simulink model "Example"  (R2016a)
settings: Solver=FixedStepAuto  StartTime=0.0  StopTime=EndTime  FixedStep=SampleTime  RelTol=1e-3
values from neighbouring files (symbols this model uses):
  A1_IC = pi/4    (= 0.785398163397)    [LaserBeamStability_CommandScript.m]
  A2_IC = pi/4    (= 0.785398163397)    [LaserBeamStability_CommandScript.m]
  A3_IC = pi/4    (= 0.785398163397)    [LaserBeamStability_CommandScript.m]
  A4_IC = pi/4    (= 0.785398163397)    [LaserBeamStability_CommandScript.m]
  ActArm = 3.85    [LaserBeamStability_CommandScript.m]
  b12 = d(14)-d(14)*d(15)/f(2)+d(15)    [LaserBeamStability_CommandScript.m]
  b34 = d(18)-(d(18)*d(19))/f(4)+d(19)    [LaserBeamStability_CommandScript.m]
  c12 = pi/2-2*Beta(2)    [LaserBeamStability_CommandScript.m]
  c34 = pi/2-2*Beta(4)    [LaserBeamStability_CommandScript.m]
  EndTime = 1    [LaserBeamStability_CommandScript.m]
  g12 = d(13)-d(13)*d(12)/f(1)+d(12)    [LaserBeamStability_CommandScript.m]
  g34 = d(17)-(d(17)*d(16))/f(3)+d(16)    [LaserBeamStability_CommandScript.m]
  h12 = pi/2-2*Beta(1)    [LaserBeamStability_CommandScript.m]
  h34 = pi/2-2*Beta(3)    [LaserBeamStability_CommandScript.m]
  n_BS = 1.52    [LaserBeamStability_CommandScript.m]
  n_FS = 1.00    (= 1)    [LaserBeamStability_CommandScript.m]
  NuetralPoint = (Maximum_Extension-Minimum_Extension)/2    (= 6.25)    [LaserBeamStability_CommandScript.m]
  Optical_Plane_1_Command = [0 0]    [LaserBeamStability_CommandScript.m]
  SampleTime = 1/10    (= 0.1)    [LaserBeamStability_CommandScript.m]
  Sensor12Matx = [a12+b12/d(6) -b12/d(6); g12/d(6) e12-g12/d(6)]    [LaserBeamStability_CommandScript.m]
  Sensor34Matx = [a34+b34/d(10) -b34/d(10); g34/d(10) e34-g34/d(10)]    [LaserBeamStability_CommandScript.m]
  SocketID = TCP_ConnectToServer(IP_ADD, Port, TimeOut)    [LaserBeamStability_CommandScript.m]
  t12 = 2.5    [LaserBeamStability_CommandScript.m]
  t34 = 2.5    [LaserBeamStability_CommandScript.m]
  Target_Command = [0 0]    [LaserBeamStability_CommandScript.m]
undefined symbols (not defined in the file or in its folder): A, Beta, D, d, f, l, positioner, Td, TLense
libraries: simulink x1
settings Model: Creator=Justin  LastModifiedBy=Justin
settings SolverCC: ZeroCrossControl=EnableAll  ZeroCrossAlgorithm=Adaptive

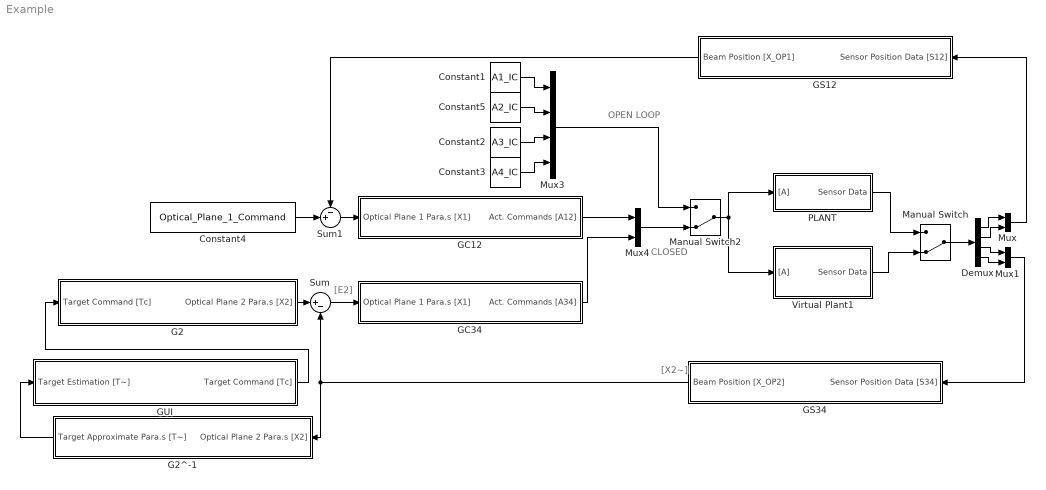
== system Example ==
  note: CLOSED
  note: OPEN LOOP
  note: [X2~]
  note: [E2]
  Constant1 : Constant  Value=A1_IC
  Constant2 : Constant  Value=A3_IC
  Constant3 : Constant  Value=A4_IC
  Constant4 : Constant  Value=Optical_Plane_1_Command
  Constant5 : Constant  Value=A2_IC
  Demux : Demux
  G2 : Subsystem
  G2^-1 : Subsystem
  GC12 : Subsystem
  GC34 : Subsystem
  GS12 : Subsystem
  GS34 : Subsystem
  GUI : Subsystem
  Manual Switch : ManualSwitch  CurrentSetting=0
  Manual Switch2 : ManualSwitch  CurrentSetting=0
  Mux : Mux  Inputs=2
  Mux1 : Mux  Inputs=2
  Mux3 : Mux
  Mux4 : Mux  Inputs=2
  PLANT : Subsystem
  Sum : Sum  Inputs=|+-
  Sum1 : Sum  Inputs=-+|
  Virtual Plant1 : Subsystem
  wires:
  G2/1(Optical Plane 2 Para.s [X2]) -> Sum/1
  G2^-1/1(Target Approximate Para.s [T~]) -> GUI/1(Target Estimation [T~])
  GUI/1(Target Command [Tc]) -> G2/1(Target Command [Tc])
  PLANT/1(Sensor Data) -> Manual Switch/1
  Demux/1 -> Mux/1
  Demux/2 -> Mux/2
  Demux/3 -> Mux1/1
  Demux/4 -> Mux1/2
  Mux/1 -> GS12/1(Sensor Position Data [S12])
  Mux1/1 -> GS34/1(Sensor Position Data [S34])
  Sum/1 -> GC34/1(Optical Plane 1 Para.s [X1])
  GC34/1(Act. Commands [A34]) -> Mux4/2
  GS34/1(Beam Position [X_OP2]) -> G2^-1/1(Optical Plane 2 Para.s [X2]), Sum/2
  Sum1/1 -> GC12/1(Optical Plane 1 Para.s [X1])
  GS12/1(Beam Position [X_OP1]) -> Sum1/1
  Constant5/1 -> Mux3/2
  Constant1/1 -> Mux3/1
  GC12/1(Act. Commands [A12]) -> Mux4/1
  Virtual Plant1/1(Sensor Data) -> Manual Switch/2
  Manual Switch/1 -> Demux/1
  Constant2/1 -> Mux3/3
  Constant3/1 -> Mux3/4
  Mux4/1 -> Manual Switch2/2
  Mux3/1 -> Manual Switch2/1
  Manual Switch2/1 -> Virtual Plant1/1("[A]"), PLANT/1("[A]")
  Constant4/1 -> Sum1/2

== system Example/G2 ==
  Target Command [Tc] : Inport
  Beam Pass 3 Inv : Subsystem
  Beam Pass 4 Inv : Subsystem
  l10 inv : Gain  Gain=([1 d(10); 0 1])^-1  Multiplication=Matrix(K*u)
  l11 inv : Gain  Gain=([1 d(11); 0 1])^-1  Multiplication=Matrix(K*u)
  l9 inv : Gain  Gain=([1 d(9); 0 1])^-1  Multiplication=Matrix(K*u)
  Optical Plane 2 Para.s [X2] : Outport
  wires:
  Target Command [Tc]/1 -> l11 inv/1
  l11 inv/1 -> Beam Pass 4 Inv/1(Passed Parameters)
  Beam Pass 4 Inv/1("Approximated Incoming Parameters ") -> l10 inv/1
  l10 inv/1 -> Beam Pass 3 Inv/1(Passed Parameters)
  Beam Pass 3 Inv/1("Approximated Incoming Parameters ") -> l9 inv/1
  l9 inv/1 -> Optical Plane 2 Para.s [X2]/1

== system Example/G2^-1 ==
  Optical Plane 2 Para.s [X2] : Inport
  Beam Pass 3 : Subsystem
  Beam Pass 4 : Subsystem
  l(10) : Gain  Gain=([1 d(10); 0 1])  Multiplication=Matrix(K*u)
  l(11) : Gain  Gain=([1 d(11); 0 1])  Multiplication=Matrix(K*u)
  l(9) : Gain  Gain=([1 d(9); 0 1])  Multiplication=Matrix(K*u)
  Target Approximate Para.s [T~] : Outport
  wires:
  Optical Plane 2 Para.s [X2]/1 -> l(9)/1
  l(11)/1 -> Target Approximate Para.s [T~]/1
  l(9)/1 -> Beam Pass 3/1(Approximated Optical Plane 2 Parameters)
  Beam Pass 3/1("Approximated Target Parameters ") -> l(10)/1
  l(10)/1 -> Beam Pass 4/1(Approximated Optical Plane 2 Parameters)
  Beam Pass 4/1("Approximated Target Parameters ") -> l(11)/1

== system Example/GC12 ==
  Optical Plane 1 Para.s [X1] : Inport
  IC2 : InitialCondition  Value=[A1_IC A2_IC]
  Sum : Sum  Inputs=|++
  Transport^-1 : Subsystem
  Unit Delay2 : UnitDelay  InitialCondition=[A1_IC A2_IC]  SampleTime=SampleTime
  "[Nu]^-1" : Subsystem
  Act. Commands [A12] : Outport
  wires:
  Optical Plane 1 Para.s [X1]/1 -> Transport^-1/1(Optical Plane 1 Para.s [X1])
  "[Nu]^-1"/1("[A_12]") -> Sum/1
  Sum/1 -> IC2/1
  Transport^-1/1("[E_A2']") -> "[Nu]^-1"/1("[E_A2']")
  IC2/1 -> Unit Delay2/1, Act. Commands [A12]/1
  Unit Delay2/1 -> "[Nu]^-1"/2("[A_12]z^-1"), Sum/2

== system Example/GC34 ==
  Optical Plane 1 Para.s [X1] : Inport
  Demux : Demux  Outputs=2
  IC2 : InitialCondition  Value=[A1_IC A2_IC]
  Mux : Mux  Inputs=2
  Sum : Sum  Inputs=|++
  Transport^-1 : Subsystem
  Unit Delay : UnitDelay  InitialCondition=A1_IC  SampleTime=SampleTime
  Unit Delay1 : UnitDelay  InitialCondition=A2_IC  SampleTime=SampleTime
  "[Nu]^-1" : Subsystem
  Act. Commands [A34] : Outport
  wires:
  IC2/1 -> Act. Commands [A34]/1, Demux/1
  Demux/2 -> Unit Delay1/1
  Demux/1 -> Unit Delay/1
  Unit Delay1/1 -> Mux/2
  Unit Delay/1 -> Mux/1
  Transport^-1/1("[E_A2']") -> "[Nu]^-1"/1("[E_A2']")
  Mux/1 -> Sum/2, "[Nu]^-1"/2("[A_12]z^-1")
  Sum/1 -> IC2/1
  "[Nu]^-1"/1("[A_12]") -> Sum/1
  Optical Plane 1 Para.s [X1]/1 -> Transport^-1/1(Optical Plane 1 Para.s [X1])

== system Example/GS12 ==
  note: Theta op1
  note: rop1
  note: R_S2
  note: R_S1
  note: rl6'
  note: rop1
  Sensor Position Data [S12] : Inport
  Constant1 : Constant  Value=b12*c12
  Constant2 : Constant  Value=d(6)
  Constant6 : Constant  Value=g12*h12
  Demux : Demux  Outputs=2
  Demux1 : Demux  Outputs=2
  Gain : Gain  Gain=Sensor12Matx^-1  Multiplication=Matrix(K*u)
  Mux : Mux  Inputs=2
  Mux1 : Mux  Inputs=2
  Product : Product  Inputs=*/
  Sum : Sum  Inputs=|+-
  Sum1 : Sum  Inputs=-+|
  Sum2 : Sum  Inputs=+-|
  Beam Position [X_OP1] : Outport
  wires:
  Product/1 -> Mux/2
  Constant2/1 -> Product/2
  Sum2/1 -> Product/1
  Demux1/1 -> Sum2/1
  Demux1/2 -> Mux/1, Sum2/2
  Sum/1 -> Mux1/2
  Sum1/1 -> Mux1/1
  Mux1/1 -> Gain/1
  Constant6/1 -> Sum/2
  Constant1/1 -> Sum1/1
  Demux/1 -> Sum/1
  Demux/2 -> Sum1/2
  Gain/1 -> Demux1/1
  Sensor Position Data [S12]/1 -> Demux/1
  Mux/1 -> Beam Position [X_OP1]/1

== system Example/GS34 ==
  note: rop2
  note: rl10'
  note: R_S3
  note: R_S4
  note: rop2
  note: Theta op2
  Sensor Position Data [S34] : Inport
  Constant1 : Constant  Value=b34*c34
  Constant2 : Constant  Value=d(10)
  Constant6 : Constant  Value=g34*h34
  Demux : Demux  Outputs=2
  Demux1 : Demux  Outputs=2
  Gain : Gain  Gain=Sensor34Matx^-1  Multiplication=Matrix(K*u)
  Mux : Mux  Inputs=2
  Mux1 : Mux  Inputs=2
  Product : Product  Inputs=*/
  Sum : Sum  Inputs=|+-
  Sum1 : Sum  Inputs=-+|
  Sum2 : Sum  Inputs=+-|
  Beam Position [X_OP2] : Outport
  wires:
  Mux/1 -> Beam Position [X_OP2]/1
  Sensor Position Data [S34]/1 -> Demux/1
  Gain/1 -> Demux1/1
  Demux/2 -> Sum1/2
  Demux/1 -> Sum/1
  Constant1/1 -> Sum1/1
  Constant6/1 -> Sum/2
  Mux1/1 -> Gain/1
  Sum1/1 -> Mux1/1
  Sum/1 -> Mux1/2
  Demux1/2 -> Sum2/2, Mux/1
  Demux1/1 -> Sum2/1
  Sum2/1 -> Product/1
  Constant2/1 -> Product/2
  Product/1 -> Mux/2

== system Example/GUI ==
  Target Estimation [T~] : Inport
  Constant : Constant  Value=Target_Command(1)
  Constant1 : Constant  Value=Target_Command(2)
  Mux : Mux  Inputs=2
  "Target Approximation Scope " : Scope
  To Workspace : ToWorkspace  VariableName=Target_Estimation  SaveFormat=Timeseries  SampleTime=-1
  Target Command [Tc] : Outport
  wires:
  Target Estimation [T~]/1 -> To Workspace/1, "Target Approximation Scope "/1
  Mux/1 -> Target Command [Tc]/1
  Constant/1 -> Mux/1
  Constant1/1 -> Mux/2

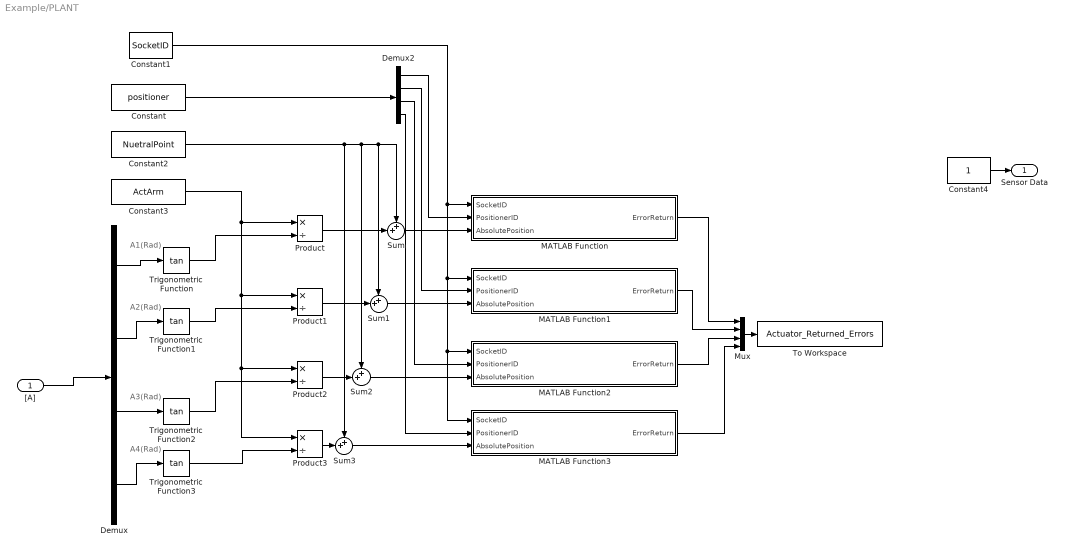
== system Example/PLANT ==
  note: A1(Rad)
  note: A2(Rad)
  note: A3(Rad)
  note: A4(Rad)
  "[A]" : Inport
  Constant : Constant  Value=positioner
  Constant1 : Constant  Value=SocketID
  Constant2 : Constant  Value=NuetralPoint
  Constant3 : Constant  Value=ActArm
  Constant4 : Constant
  Demux : Demux
  Demux2 : Demux
  MATLAB Function : MATLAB Function  TreatAsAtomicUnit=on
  MATLAB Function1 : MATLAB Function  TreatAsAtomicUnit=on
  MATLAB Function2 : MATLAB Function  TreatAsAtomicUnit=on
  MATLAB Function3 : MATLAB Function  TreatAsAtomicUnit=on
  Mux : Mux
  Product{,1..3} (4 alike) : Product  Inputs=*/
  Sum{,1..3} (4 alike) : Sum  Inputs=++|
  To Workspace : ToWorkspace  VariableName=Actuator_Returned_Errors  SaveFormat=Timeseries  SampleTime=-1
  Trigonometric Function{,1..3} (4 alike) : Trigonometry  Operator=tan
  Sensor Data : Outport
  wires:
  "[A]"/1 -> Demux/1
  Constant/1 -> Demux2/1
  Demux2/1 -> MATLAB Function/2(PositionerID)
  Demux2/2 -> MATLAB Function1/2(PositionerID)
  Demux2/3 -> MATLAB Function2/2(PositionerID)
  Demux2/4 -> MATLAB Function3/2(PositionerID)
  Constant1/1 -> MATLAB Function3/1(SocketID), MATLAB Function2/1(SocketID), MATLAB Function1/1(SocketID), MATLAB Function/1(SocketID)
  Sum/1 -> MATLAB Function/3(AbsolutePosition)
  Demux/1 -> Trigonometric Function/1
  Demux/2 -> Trigonometric Function1/1
  Demux/4 -> Trigonometric Function3/1
  Product/1 -> Sum/2
  Product1/1 -> Sum1/2
  Sum1/1 -> MATLAB Function1/3(AbsolutePosition)
  Constant2/1 -> Sum2/1, Sum1/1, Sum/1, Sum3/1
  Sum2/1 -> MATLAB Function2/3(AbsolutePosition)
  Sum3/1 -> MATLAB Function3/3(AbsolutePosition)
  Product3/1 -> Sum3/2
  Product2/1 -> Sum2/2
  Constant3/1 -> Product3/1, Product2/1, Product1/1, Product/1
  Trigonometric Function3/1 -> Product3/2
  Trigonometric Function2/1 -> Product2/2
  Trigonometric Function1/1 -> Product1/2
  Trigonometric Function/1 -> Product/2
  Mux/1 -> To Workspace/1
  MATLAB Function/1(ErrorReturn) -> Mux/1
  MATLAB Function1/1(ErrorReturn) -> Mux/2
  MATLAB Function2/1(ErrorReturn) -> Mux/3
  MATLAB Function3/1(ErrorReturn) -> Mux/4
  Constant4/1 -> Sensor Data/1
  Demux/3 -> Trigonometric Function2/1

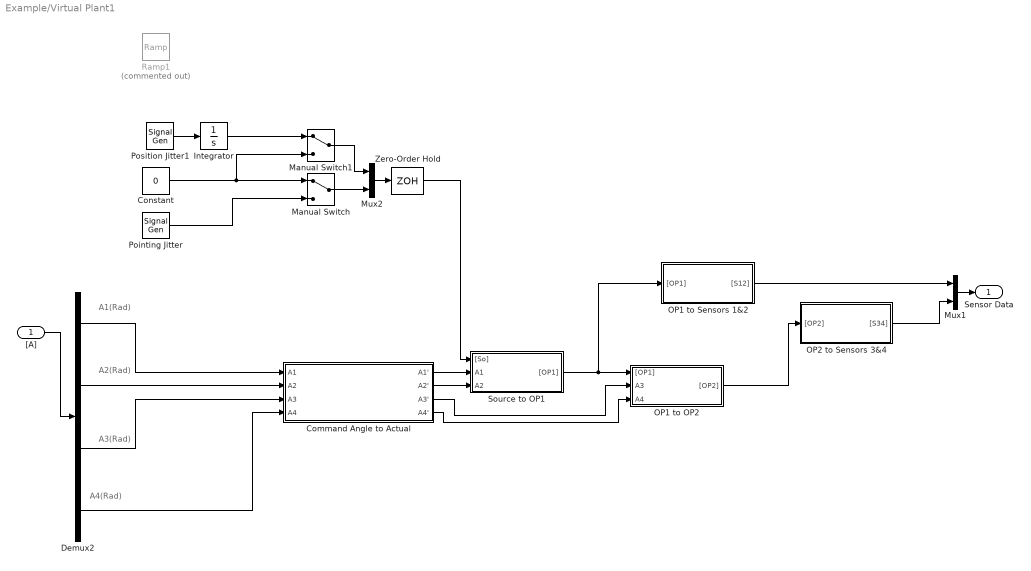
== system Example/Virtual Plant1 ==
  note: A4(Rad)
  note: A3(Rad)
  note: A2(Rad)
  note: A1(Rad)
  "[A]" : Inport
  Command Angle to Actual : Subsystem
  Constant : Constant  Value=0
  Demux2 : Demux
  Integrator : Integrator
  Manual Switch : ManualSwitch
  Manual Switch1 : ManualSwitch
  Mux1 : Mux  Inputs=2
  Mux2 : Mux  Inputs=2
  OP1 to OP2 : Subsystem
  OP1 to Sensors 1&2 : Subsystem
  OP2 to Sensors 3&4 : Subsystem
  Pointing Jitter : SignalGenerator  Amplitude=0.001  Frequency=1/EndTime
  Position Jitter1 : SignalGenerator  WaveForm=random  Amplitude=-0.5  Frequency=5/EndTime
  Ramp1 : simulink/Sources/Ramp  Commented=on  slope=A/EndTime  start=0  X0=0
  Source to OP1 : Subsystem
  Zero-Order Hold : ZeroOrderHold  SampleTime=SampleTime
  Sensor Data : Outport
  wires:
  Pointing Jitter/1 -> Manual Switch/2
  Constant/1 -> Manual Switch1/2, Manual Switch/1
  Manual Switch1/1 -> Mux2/1
  Manual Switch/1 -> Mux2/2
  Mux2/1 -> Zero-Order Hold/1
  OP2 to Sensors 3&4/1("[S34]") -> Mux1/2
  OP1 to OP2/1("[OP2]") -> OP2 to Sensors 3&4/1("[OP2]")
  OP1 to Sensors 1&2/1("[S12]") -> Mux1/1
  Mux1/1 -> Sensor Data/1
  Source to OP1/1("[OP1]") -> OP1 to OP2/1("[OP1]"), OP1 to Sensors 1&2/1("[OP1]")
  Command Angle to Actual/1(A1') -> Source to OP1/2(A1)
  Command Angle to Actual/2(A2') -> Source to OP1/3(A2)
  Command Angle to Actual/3(A3') -> OP1 to OP2/2(A3)
  Command Angle to Actual/4(A4') -> OP1 to OP2/3(A4)
  Demux2/1 -> Command Angle to Actual/1(A1)
  Demux2/2 -> Command Angle to Actual/2(A2)
  Demux2/3 -> Command Angle to Actual/3(A3)
  Demux2/4 -> Command Angle to Actual/4(A4)
  "[A]"/1 -> Demux2/1
  Zero-Order Hold/1 -> Source to OP1/1("[So]")
  Position Jitter1/1 -> Integrator/1
  Integrator/1 -> Manual Switch1/1

== system Example/G2/Beam Pass 3 Inv ==
  note: r'
  note: theta'
  note: r
  note: Theta
  Passed Parameters : Inport
  Demux : Demux  Outputs=2
  Mux : Mux  Inputs=2
  Sine : Trigonometry
  Snell Ratio : Gain  Gain=n_FS/n_BS  Multiplication=Matrix(K*u)
  Sum : Sum  Inputs=|+-
  Sum1 : Sum  Inputs=|+-
  Tangent : Trigonometry  Operator=tan
  Thickness Offset 1 : Gain  Gain=D(3)*cos(Beta(3))
  Thickness Offset 2 : Constant  Value=D(3)*sin(Beta(3))
  "Approximated Incoming Parameters " : Outport
  wires:
  Thickness Offset 2/1 -> Sum1/2
  Thickness Offset 1/1 -> Sum1/1
  Tangent/1 -> Thickness Offset 1/1
  Snell Ratio/1 -> Tangent/1
  Sine/1 -> Snell Ratio/1
  Demux/1 -> Sum/1
  Demux/2 -> Sine/1, Mux/2
  Sum/1 -> Mux/1
  Mux/1 -> "Approximated Incoming Parameters "/1
  Sum1/1 -> Sum/2
  Passed Parameters/1 -> Demux/1

== system Example/G2/Beam Pass 4 Inv ==
  note: Theta
  note: r
  note: theta'
  note: r'
  Passed Parameters : Inport
  Demux : Demux  Outputs=2
  Mux : Mux  Inputs=2
  Sine : Trigonometry
  Snell Ratio : Gain  Gain=n_FS/n_BS
  Sum : Sum  Inputs=|+-
  Sum1 : Sum  Inputs=|+-
  Tangent : Trigonometry  Operator=tan
  Thickness Offset 1 : Gain  Gain=D(4)*cos(Beta(4))
  Thickness Offset 2 : Constant  Value=D(4)*sin(Beta(4))
  "Approximated Incoming Parameters " : Outport
  wires:
  Passed Parameters/1 -> Demux/1
  Sum1/1 -> Sum/2
  Mux/1 -> "Approximated Incoming Parameters "/1
  Sum/1 -> Mux/1
  Demux/2 -> Mux/2, Sine/1
  Demux/1 -> Sum/1
  Sine/1 -> Snell Ratio/1
  Snell Ratio/1 -> Tangent/1
  Tangent/1 -> Thickness Offset 1/1
  Thickness Offset 1/1 -> Sum1/1
  Thickness Offset 2/1 -> Sum1/2

== system Example/G2^-1/Beam Pass 3 ==
  Approximated Optical Plane 2 Parameters : Inport
  Demux : Demux  Outputs=2
  Mux : Mux  Inputs=2
  Sine : Trigonometry
  Snell Ratio : Gain  Gain=n_FS/n_BS
  Sum : Sum  Inputs=|++
  Sum1 : Sum  Inputs=|+-
  Tangent : Trigonometry  Operator=tan
  Thickness Offset 1 : Gain  Gain=D(3)*cos(Beta(3))
  Thickness Offset 2 : Constant  Value=D(3)*sin(Beta(3))
  "Approximated Target Parameters " : Outport
  wires:
  Approximated Optical Plane 2 Parameters/1 -> Demux/1
  Mux/1 -> "Approximated Target Parameters "/1
  Demux/1 -> Sum/1
  Sum/1 -> Mux/1
  Sum1/1 -> Sum/2
  Demux/2 -> Sine/1, Mux/2
  Snell Ratio/1 -> Tangent/1
  Sine/1 -> Snell Ratio/1
  Tangent/1 -> Thickness Offset 1/1
  Thickness Offset 1/1 -> Sum1/1
  Thickness Offset 2/1 -> Sum1/2

== system Example/G2^-1/Beam Pass 4 ==
  Approximated Optical Plane 2 Parameters : Inport
  Demux : Demux  Outputs=2
  Mux : Mux  Inputs=2
  Sine : Trigonometry
  Snell Ratio : Gain  Gain=n_FS/n_BS
  Sum : Sum  Inputs=|++
  Sum1 : Sum  Inputs=|+-
  Tangent : Trigonometry  Operator=tan
  Thickness Offset 1 : Gain  Gain=D(4)*cos(Beta(4))
  Thickness Offset 2 : Constant  Value=D(4)*sin(Beta(4))
  "Approximated Target Parameters " : Outport
  wires:
  Thickness Offset 2/1 -> Sum1/2
  Thickness Offset 1/1 -> Sum1/1
  Tangent/1 -> Thickness Offset 1/1
  Sine/1 -> Snell Ratio/1
  Snell Ratio/1 -> Tangent/1
  Demux/2 -> Mux/2, Sine/1
  Sum1/1 -> Sum/2
  Sum/1 -> Mux/1
  Demux/1 -> Sum/1
  Mux/1 -> "Approximated Target Parameters "/1
  Approximated Optical Plane 2 Parameters/1 -> Demux/1

== system Example/GC12/Transport^-1 ==
  Optical Plane 1 Para.s [X1] : Inport
  (Four Box Transfer)^-1 : Subsystem
  l(3)^-1 : Gain  Gain=([1 d(3); 0 1])^-1  Multiplication=Matrix(K*u)
  l(5)^-1 : Gain  Gain=([1 d(5); 0 1])^-1  Multiplication=Matrix(K*u)
  "[E_A2']" : Outport
  wires:
  Optical Plane 1 Para.s [X1]/1 -> l(5)^-1/1
  l(5)^-1/1 -> (Four Box Transfer)^-1/1(Beam Para.s Out of Transport)
  (Four Box Transfer)^-1/1(Beam Para.s into Transport) -> l(3)^-1/1
  l(3)^-1/1 -> "[E_A2']"/1

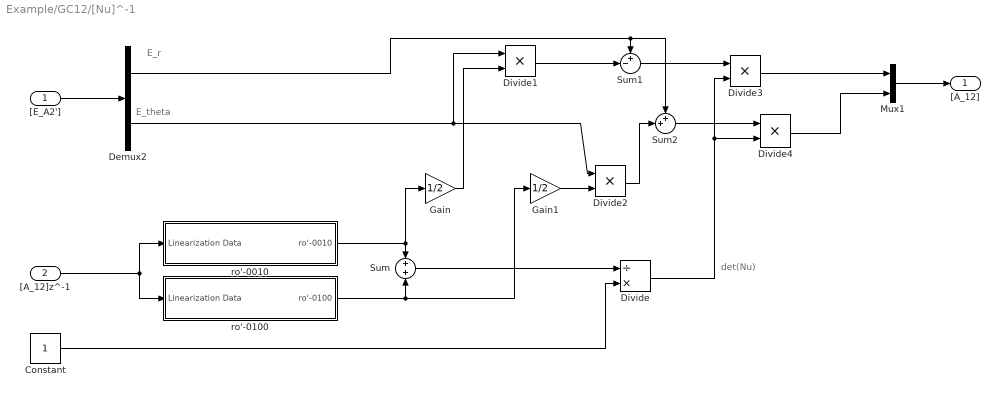
== system Example/GC12/[Nu]^-1 ==
  note: det(Nu)
  note: E_theta
  note: E_r
  "[E_A2']" : Inport
  "[A_12]z^-1" : Inport  Port=2
  Constant : Constant
  Demux2 : Demux  Outputs=2
  Divide : Product  Inputs=/*
  Divide{1..4} (4 alike) : Product  Inputs=**
  Gain : Gain  Gain=1/2
  Gain1 : Gain  Gain=1/2
  Mux1 : Mux  Inputs=2
  Sum : Sum  Inputs=+|+
  Sum1 : Sum  Inputs=+-|
  Sum2 : Sum  Inputs=++|
  ro'-0010 : Subsystem
  "ro'-0100 " : Subsystem
  "[A_12]" : Outport
  wires:
  "[A_12]z^-1"/1 -> ro'-0010/1(Linearization Data), "ro'-0100 "/1(Linearization Data)
  ro'-0010/1(ro'-0010) -> Gain/1, Sum/1
  "ro'-0100 "/1(ro'-0100) -> Gain1/1, Sum/2
  Sum/1 -> Divide/1
  Constant/1 -> Divide/2
  Mux1/1 -> "[A_12]"/1
  Divide3/1 -> Mux1/1
  Divide4/1 -> Mux1/2
  Divide/1 -> Divide3/2, Divide4/2
  "[E_A2']"/1 -> Demux2/1
  Sum1/1 -> Divide3/1
  Demux2/1 -> Sum2/1, Sum1/1
  Gain/1 -> Divide1/2
  Divide1/1 -> Sum1/2
  Sum2/1 -> Divide4/1
  Gain1/1 -> Divide2/2
  Divide2/1 -> Sum2/2
  Demux2/2 -> Divide2/1, Divide1/1

== system Example/GC34/Transport^-1 ==
  Optical Plane 1 Para.s [X1] : Inport
  (Four Box Transfer)^-1 : Subsystem
  l(3)^-1 : Gain  Gain=([1 d(3); 0 1])^-1  Multiplication=Matrix(K*u)
  l(5)^-1 : Gain  Gain=([1 d(5); 0 1])^-1  Multiplication=Matrix(K*u)
  "[E_A2']" : Outport
  wires:
  l(3)^-1/1 -> "[E_A2']"/1
  (Four Box Transfer)^-1/1(Beam Para.s into Transport) -> l(3)^-1/1
  l(5)^-1/1 -> (Four Box Transfer)^-1/1(Beam Para.s Out of Transport)
  Optical Plane 1 Para.s [X1]/1 -> l(5)^-1/1

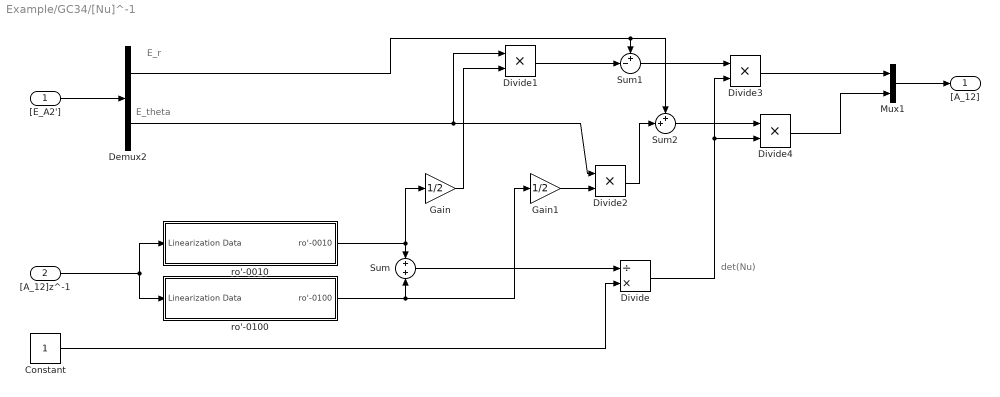
== system Example/GC34/[Nu]^-1 ==
  note: E_r
  note: E_theta
  note: det(Nu)
  "[E_A2']" : Inport
  "[A_12]z^-1" : Inport  Port=2
  Constant : Constant
  Demux2 : Demux  Outputs=2
  Divide : Product  Inputs=/*
  Divide{1..4} (4 alike) : Product  Inputs=**
  Gain : Gain  Gain=1/2
  Gain1 : Gain  Gain=1/2
  Mux1 : Mux  Inputs=2
  Sum : Sum  Inputs=+|+
  Sum1 : Sum  Inputs=+-|
  Sum2 : Sum  Inputs=++|
  ro'-0010 : Subsystem
  "ro'-0100 " : Subsystem
  "[A_12]" : Outport
  wires:
  Demux2/2 -> Divide1/1, Divide2/1
  Divide2/1 -> Sum2/2
  Gain1/1 -> Divide2/2
  Sum2/1 -> Divide4/1
  Divide1/1 -> Sum1/2
  Gain/1 -> Divide1/2
  Demux2/1 -> Sum1/1, Sum2/1
  Sum1/1 -> Divide3/1
  "[E_A2']"/1 -> Demux2/1
  Divide/1 -> Divide4/2, Divide3/2
  Divide4/1 -> Mux1/2
  Divide3/1 -> Mux1/1
  Mux1/1 -> "[A_12]"/1
  Constant/1 -> Divide/2
  Sum/1 -> Divide/1
  "ro'-0100 "/1(ro'-0100) -> Sum/2, Gain1/1
  ro'-0010/1(ro'-0010) -> Sum/1, Gain/1
  "[A_12]z^-1"/1 -> "ro'-0100 "/1(Linearization Data), ro'-0010/1(Linearization Data)

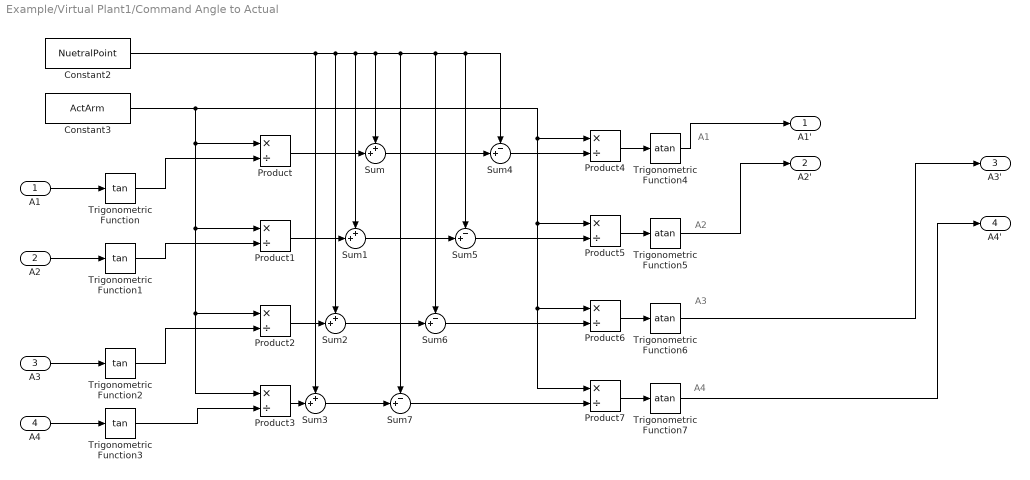
== system Example/Virtual Plant1/Command Angle to Actual ==
  note: A1
  note: A2
  note: A3
  note: A4
  A1 : Inport
  A2 : Inport  Port=2
  A3 : Inport  Port=3
  A4 : Inport  Port=4
  Constant2 : Constant  Value=NuetralPoint
  Constant3 : Constant  Value=ActArm
  Product{,1..7} (8 alike) : Product  Inputs=*/
  Sum{,1..3} (4 alike) : Sum  Inputs=++|
  Sum{4..7} (4 alike) : Sum  Inputs=-+|
  Trigonometric Function{,1..3} (4 alike) : Trigonometry  Operator=tan
  Trigonometric Function{4..7} (4 alike) : Trigonometry  Operator=atan
  A1' : Outport
  A2' : Outport  Port=2
  A3' : Outport  Port=3
  A4' : Outport  Port=4
  wires:
  Product4/1 -> Trigonometric Function4/1
  Trigonometric Function6/1 -> A3'/1
  Sum2/1 -> Sum6/2
  Product7/1 -> Trigonometric Function7/1
  Product6/1 -> Trigonometric Function6/1
  Product3/1 -> Sum3/2
  Constant3/1 -> Product4/1, Product5/1, Product6/1, Product7/1, Product/1, Product1/1, Product2/1, Product3/1
  A3/1 -> Trigonometric Function2/1
  Product1/1 -> Sum1/2
  A2/1 -> Trigonometric Function1/1
  Trigonometric Function2/1 -> Product2/2
  A1/1 -> Trigonometric Function/1
  Trigonometric Function1/1 -> Product1/2
  Constant2/1 -> Sum3/1, Sum/1, Sum7/1, Sum6/1, Sum5/1, Sum4/1, Sum1/1, Sum2/1
  Product/1 -> Sum/2
  Trigonometric Function/1 -> Product/2
  A4/1 -> Trigonometric Function3/1
  Product2/1 -> Sum2/2
  Trigonometric Function3/1 -> Product3/2
  Sum1/1 -> Sum5/2
  Sum5/1 -> Product5/2
  Sum4/1 -> Product4/2
  Sum3/1 -> Sum7/2
  Sum7/1 -> Product7/2
  Sum6/1 -> Product6/2
  Trigonometric Function7/1 -> A4'/1
  Trigonometric Function5/1 -> A2'/1
  Trigonometric Function4/1 -> A1'/1
  Product5/1 -> Trigonometric Function5/1
  Sum/1 -> Sum4/2

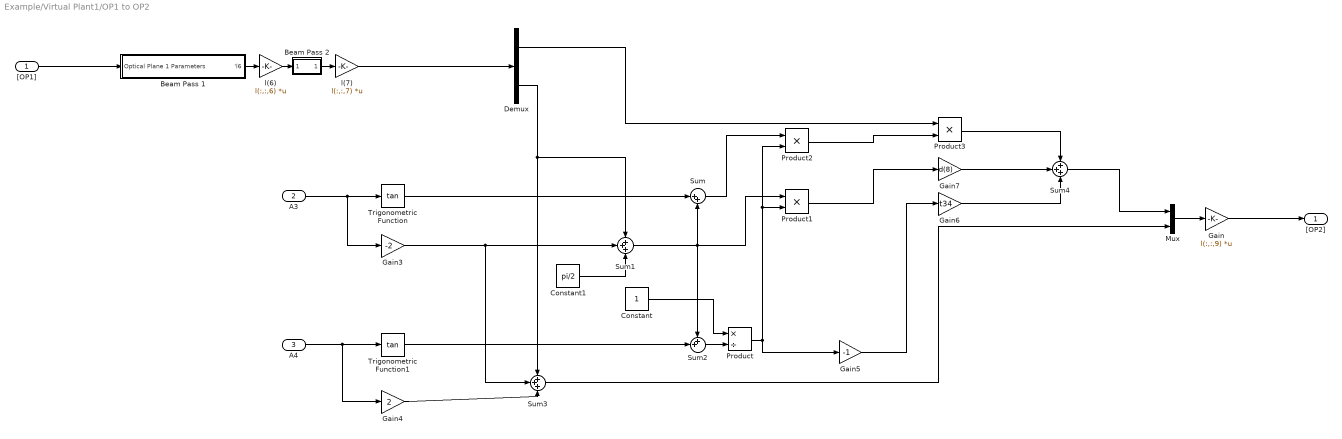
== system Example/Virtual Plant1/OP1 to OP2 ==
  "[OP1]" : Inport
  A3 : Inport  Port=2
  A4 : Inport  Port=3
  Beam Pass 1 : Subsystem
  Beam Pass 2 : Subsystem
  Constant : Constant
  Constant1 : Constant  Value=pi/2
  Demux : Demux  Outputs=2
  Gain : Gain  Gain=l(:,:,9)  Multiplication=Matrix(K*u)
  Gain3 : Gain  Gain=-2
  Gain4 : Gain  Gain=2
  Gain5 : Gain  Gain=-1
  Gain6 : Gain  Gain=t34
  Gain7 : Gain  Gain=d(8)
  Mux : Mux  Inputs=2
  Product : Product  Inputs=*/
  Product1 : Product  Inputs=**
  Product2 : Product  Inputs=**
  Product3 : Product  Inputs=**
  Sum : Sum  Inputs=|++
  Sum1 : Sum  Inputs=+++
  Sum2 : Sum  Inputs=++|
  Sum3 : Sum  Inputs=+++
  Sum4 : Sum  Inputs=+++
  Trigonometric Function : Trigonometry  Operator=tan
  Trigonometric Function1 : Trigonometry  Operator=tan
  l(6) : Gain  Gain=l(:,:,6)  Multiplication=Matrix(K*u)
  l(7) : Gain  Gain=l(:,:,7)  Multiplication=Matrix(K*u)
  "[OP2]" : Outport
  wires:
  Constant/1 -> Product/1
  Sum2/1 -> Product/2
  l(7)/1 -> Demux/1
  "[OP1]"/1 -> Beam Pass 1/1(Optical Plane 1 Parameters)
  l(6)/1 -> Beam Pass 2/1(l6')
  Beam Pass 1/1('l6) -> l(6)/1
  Gain/1 -> "[OP2]"/1
  A4/1 -> Trigonometric Function1/1, Gain4/1
  Sum4/1 -> Mux/1
  Product3/1 -> Sum4/1
  Gain7/1 -> Sum4/2
  Gain6/1 -> Sum4/3
  Gain5/1 -> Gain6/1
  Product1/1 -> Gain7/1
  Demux/1 -> Product3/1
  Product2/1 -> Product3/2
  Sum/1 -> Product2/1
  Product/1 -> Product1/2, Product2/2, Gain5/1
  Sum3/1 -> Mux/2
  Gain4/1 -> Sum3/3
  Trigonometric Function1/1 -> Sum2/2
  Demux/2 -> Sum1/1, Sum3/1
  Gain3/1 -> Sum1/2, Sum3/2
  Sum1/1 -> Sum2/1, Product1/1, Sum/2
  Trigonometric Function/1 -> Sum/1
  A3/1 -> Trigonometric Function/1, Gain3/1
  Mux/1 -> Gain/1
  Beam Pass 2/1('l7) -> l(7)/1
  Constant1/1 -> Sum1/3

== system Example/Virtual Plant1/OP1 to Sensors 1&2 ==
  "[OP1]" : Inport
  Beam Reflection 1 : Subsystem
  Beam Reflection 2 : Subsystem
  Demux : Demux  Outputs=2
  Demux1 : Demux  Outputs=2
  Gain : Gain  Gain=l(:,:,6)  Multiplication=Matrix(K*u)
  Gain1 : Gain  Gain=l(12)  Multiplication=Matrix(K*u)
  Gain2 : Gain  Gain=[1 0; 1/f(1) 1]  Multiplication=Matrix(K*u)
  Gain3 : Gain  Gain=l(13)  Multiplication=Matrix(K*u)
  Gain4 : Gain  Gain=l(:,:,14)  Multiplication=Matrix(K*u)
  Gain5 : Gain  Gain=[1 0; 1/f(2) 1]  Multiplication=Matrix(K*u)
  Gain6 : Gain  Gain=l(:,:,15)  Multiplication=Matrix(K*u)
  Mux : Mux  Inputs=2
  Terminator : Terminator
  Terminator2 : Terminator
  "[S12]" : Outport
  wires:
  Demux/1 -> Mux/1
  Demux1/1 -> Mux/2
  Demux/2 -> Terminator2/1
  Demux1/2 -> Terminator/1
  Mux/1 -> "[S12]"/1
  Gain6/1 -> Demux1/1
  Gain3/1 -> Demux/1
  Gain5/1 -> Gain6/1
  Gain4/1 -> Gain5/1
  Beam Reflection 2/1(Reflected Beam) -> Gain4/1
  Gain2/1 -> Gain3/1
  Gain1/1 -> Gain2/1
  Beam Reflection 1/1(Reflected Beam) -> Gain1/1
  Gain/1 -> Beam Reflection 2/1("[OP1]")
  "[OP1]"/1 -> Gain/1, Beam Reflection 1/1("[OP1]")

== system Example/Virtual Plant1/OP2 to Sensors 3&4 ==
  "[OP2]" : Inport
  Beam Reflection 3 : Subsystem
  Beam Reflection 4 : Subsystem
  Demux : Demux  Outputs=2
  Demux1 : Demux  Outputs=2
  Gain : Gain  Gain=l(:,:,9)  Multiplication=Matrix(K*u)
  Gain1 : Gain  Gain=l(:,:,16)  Multiplication=Matrix(K*u)
  Gain2 : Gain  Gain=[1 0; 1/f(3) 1]  Multiplication=Matrix(K*u)
  Gain3 : Gain  Gain=l(:,:,17)  Multiplication=Matrix(K*u)
  Gain4 : Gain  Gain=l(:,:,18)  Multiplication=Matrix(K*u)
  Gain5 : Gain  Gain=[1 0; 1/f(4) 1]  Multiplication=Matrix(K*u)
  Gain6 : Gain  Gain=l(:,:,19)  Multiplication=Matrix(K*u)
  Mux : Mux  Inputs=2
  Terminator : Terminator
  Terminator2 : Terminator
  "[S34]" : Outport
  wires:
  Demux/1 -> Mux/1
  Demux1/1 -> Mux/2
  Demux/2 -> Terminator2/1
  Demux1/2 -> Terminator/1
  Mux/1 -> "[S34]"/1
  Gain6/1 -> Demux1/1
  Gain3/1 -> Demux/1
  Gain5/1 -> Gain6/1
  Gain4/1 -> Gain5/1
  Beam Reflection 4/1(Reflected Beam) -> Gain4/1
  Gain2/1 -> Gain3/1
  Gain1/1 -> Gain2/1
  Beam Reflection 3/1(Reflected Beam) -> Gain1/1
  Gain/1 -> Beam Reflection 4/1("[OP2]*l(9)")
  "[OP2]"/1 -> Gain/1, Beam Reflection 3/1("[OP2]")

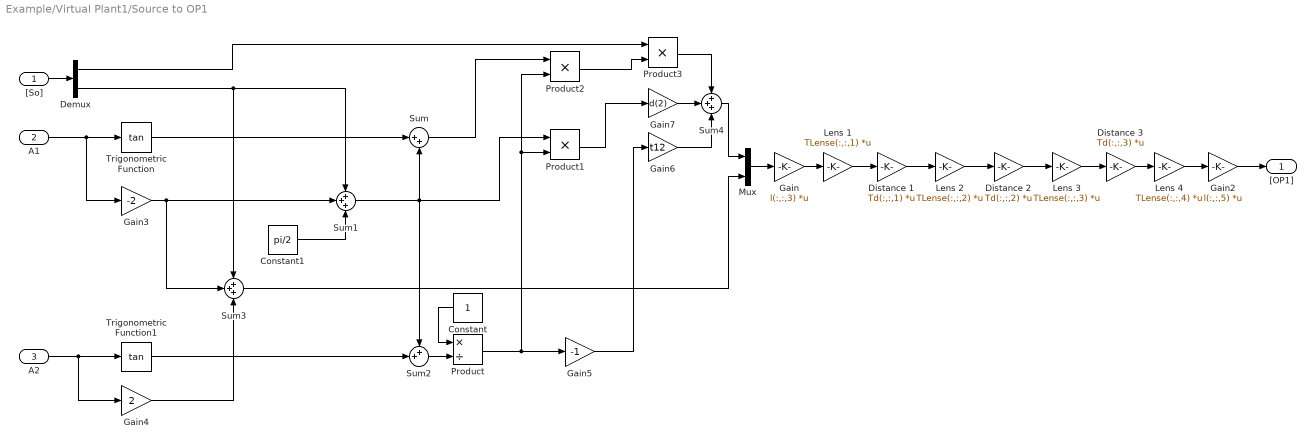
== system Example/Virtual Plant1/Source to OP1 ==
  "[So]" : Inport
  A1 : Inport  Port=2  OutMin=[pi/6]
  A2 : Inport  Port=3  OutMin=[pi/6]
  Constant : Constant
  Constant1 : Constant  Value=pi/2
  Demux : Demux  Outputs=2
  Distance 1 : Gain  Gain=Td(:,:,1)  Multiplication=Matrix(K*u)
  Distance 2 : Gain  Gain=Td(:,:,2)  Multiplication=Matrix(K*u)
  Distance 3 : Gain  Gain=Td(:,:,3)  Multiplication=Matrix(K*u)
  Gain : Gain  Gain=l(:,:,3)  Multiplication=Matrix(K*u)
  Gain2 : Gain  Gain=l(:,:,5)  Multiplication=Matrix(K*u)
  Gain3 : Gain  Gain=-2
  Gain4 : Gain  Gain=2
  Gain5 : Gain  Gain=-1
  Gain6 : Gain  Gain=t12
  Gain7 : Gain  Gain=d(2)
  Lens 1 : Gain  Gain=TLense(:,:,1)  Multiplication=Matrix(K*u)
  Lens 2 : Gain  Gain=TLense(:,:,2)  Multiplication=Matrix(K*u)
  Lens 3 : Gain  Gain=TLense(:,:,3)  Multiplication=Matrix(K*u)
  Lens 4 : Gain  Gain=TLense(:,:,4)  Multiplication=Matrix(K*u)
  Mux : Mux  Inputs=2
  Product : Product  Inputs=*/
  Product1 : Product  Inputs=**
  Product2 : Product  Inputs=**
  Product3 : Product  Inputs=**
  Sum : Sum  Inputs=|++
  Sum1 : Sum  Inputs=+++
  Sum2 : Sum  Inputs=++|
  Sum3 : Sum  Inputs=+++
  Sum4 : Sum  Inputs=+++
  Trigonometric Function : Trigonometry  Operator=tan
  Trigonometric Function1 : Trigonometry  Operator=tan
  "[OP1]" : Outport
  wires:
  Constant1/1 -> Sum1/3
  Distance 3/1 -> Lens 4/1
  Lens 4/1 -> Gain2/1
  Gain/1 -> Lens 1/1
  Lens 1/1 -> Distance 1/1
  Distance 1/1 -> Lens 2/1
  Lens 2/1 -> Distance 2/1
  Distance 2/1 -> Lens 3/1
  Lens 3/1 -> Distance 3/1
  Sum4/1 -> Mux/1
  Product3/1 -> Sum4/1
  Gain7/1 -> Sum4/2
  Gain6/1 -> Sum4/3
  Gain5/1 -> Gain6/1
  Product1/1 -> Gain7/1
  Demux/1 -> Product3/1
  Product2/1 -> Product3/2
  Sum/1 -> Product2/1
  Product/1 -> Product1/2, Product2/2, Gain5/1
  Constant/1 -> Product/1
  Sum2/1 -> Product/2
  Sum3/1 -> Mux/2
  Gain4/1 -> Sum3/3
  Trigonometric Function1/1 -> Sum2/2
  Demux/2 -> Sum1/1, Sum3/1
  Gain3/1 -> Sum1/2, Sum3/2
  Sum1/1 -> Product1/1, Sum/2, Sum2/1
  Trigonometric Function/1 -> Sum/1
  A2/1 -> Trigonometric Function1/1, Gain4/1
  A1/1 -> Trigonometric Function/1, Gain3/1
  Gain2/1 -> "[OP1]"/1
  "[So]"/1 -> Demux/1
  Mux/1 -> Gain/1

== system Example/GC12/Transport^-1/(Four Box Transfer)^-1 ==
  Beam Para.s Out of Transport : Inport
  Distance 1 : Gain  Gain=Td(:,:,1)^-1  Multiplication=Matrix(K*u)
  Distance 2 : Gain  Gain=Td(:,:,2)^-1  Multiplication=Matrix(K*u)
  Distance 3 : Gain  Gain=Td(:,:,3)^-1  Multiplication=Matrix(K*u)
  Lens 1 : Gain  Gain=TLense(:,:,1)^-1  Multiplication=Matrix(K*u)
  Lens 2 : Gain  Gain=TLense(:,:,2)^-1  Multiplication=Matrix(K*u)
  Lens 3 : Gain  Gain=TLense(:,:,3)^-1  Multiplication=Matrix(K*u)
  Lens 4 : Gain  Gain=TLense(:,:,4)^-1  Multiplication=Matrix(K*u)
  Beam Para.s into Transport : Outport
  wires:
  Beam Para.s Out of Transport/1 -> Lens 4/1
  Lens 4/1 -> Distance 3/1
  Distance 3/1 -> Lens 3/1
  Lens 3/1 -> Distance 2/1
  Distance 2/1 -> Lens 2/1
  Lens 2/1 -> Distance 1/1
  Distance 1/1 -> Lens 1/1
  Lens 1/1 -> Beam Para.s into Transport/1

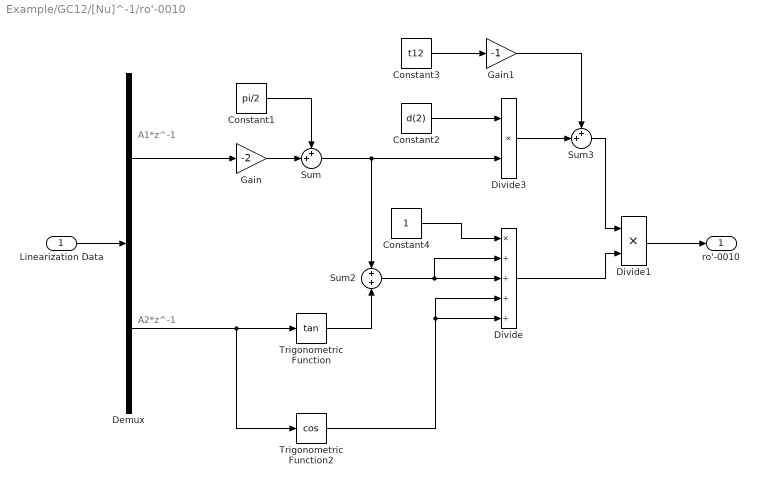
== system Example/GC12/[Nu]^-1/ro'-0010 ==
  note: A2*z^-1
  note: A1*z^-1
  Linearization Data : Inport
  Constant1 : Constant  Value=pi/2
  Constant2 : Constant  Value=d(2)
  Constant3 : Constant  Value=t12
  Constant4 : Constant
  Demux : Demux  Outputs=2
  Divide : Product  Inputs=*////
  Divide1 : Product  Inputs=**
  Divide3 : Product  Inputs=**
  Gain : Gain  Gain=-2
  Gain1 : Gain  Gain=-1
  Sum : Sum  Inputs=++|
  Sum2 : Sum  Inputs=+|+
  Sum3 : Sum  Inputs=++|
  Trigonometric Function : Trigonometry  Operator=tan
  Trigonometric Function2 : Trigonometry  Operator=cos
  ro'-0010 : Outport
  wires:
  Linearization Data/1 -> Demux/1
  Demux/1 -> Gain/1
  Gain/1 -> Sum/2
  Constant1/1 -> Sum/1
  Sum/1 -> Sum2/1, Divide3/2
  Trigonometric Function/1 -> Sum2/2
  Demux/2 -> Trigonometric Function2/1, Trigonometric Function/1
  Sum2/1 -> Divide/2, Divide/3
  Divide1/1 -> ro'-0010/1
  Divide/1 -> Divide1/2
  Constant2/1 -> Divide3/1
  Constant3/1 -> Gain1/1
  Gain1/1 -> Sum3/1
  Divide3/1 -> Sum3/2
  Sum3/1 -> Divide1/1
  Trigonometric Function2/1 -> Divide/4, Divide/5
  Constant4/1 -> Divide/1

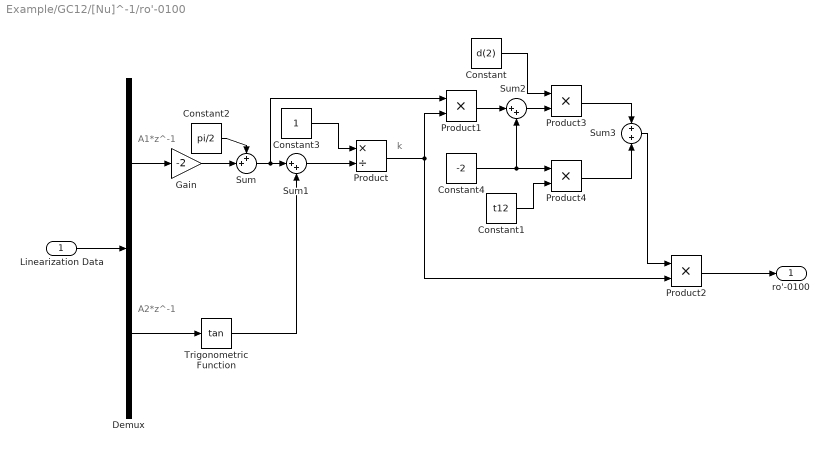
== system Example/GC12/[Nu]^-1/ro'-0100  ==
  note: k
  note: A2*z^-1
  note: A1*z^-1
  Linearization Data : Inport
  Constant : Constant  Value=d(2)
  Constant1 : Constant  Value=t12
  Constant2 : Constant  Value=pi/2
  Constant3 : Constant
  Constant4 : Constant  Value=-2
  Demux : Demux  Outputs=2
  Gain : Gain  Gain=-2
  Product : Product  Inputs=*/
  Product{1..4} (4 alike) : Product  Inputs=**
  Sum : Sum  Inputs=++|
  Sum1 : Sum  Inputs=|++
  Sum2 : Sum  Inputs=|++
  Sum3 : Sum  Inputs=+|+
  Trigonometric Function : Trigonometry  Operator=tan
  ro'-0100 : Outport
  wires:
  Linearization Data/1 -> Demux/1
  Constant2/1 -> Sum/1
  Demux/1 -> Gain/1
  Gain/1 -> Sum/2
  Demux/2 -> Trigonometric Function/1
  Trigonometric Function/1 -> Sum1/2
  Constant3/1 -> Product/1
  Product/1 -> Product1/2, Product2/2
  Sum/1 -> Product1/1, Sum1/1
  Sum1/1 -> Product/2
  Product1/1 -> Sum2/1
  Constant4/1 -> Product4/1, Sum2/2
  Sum2/1 -> Product3/2
  Constant/1 -> Product3/1
  Constant1/1 -> Product4/2
  Product4/1 -> Sum3/2
  Product3/1 -> Sum3/1
  Sum3/1 -> Product2/1
  Product2/1 -> ro'-0100/1

== system Example/GC34/Transport^-1/(Four Box Transfer)^-1 ==
  Beam Para.s Out of Transport : Inport
  Distance 1 : Gain  Gain=Td(:,:,1)^-1  Multiplication=Matrix(K*u)
  Distance 2 : Gain  Gain=Td(:,:,2)^-1  Multiplication=Matrix(K*u)
  Distance 3 : Gain  Gain=Td(:,:,3)^-1  Multiplication=Matrix(K*u)
  Lens 1 : Gain  Gain=TLense(:,:,1)^-1  Multiplication=Matrix(K*u)
  Lens 2 : Gain  Gain=TLense(:,:,2)^-1  Multiplication=Matrix(K*u)
  Lens 3 : Gain  Gain=TLense(:,:,3)^-1  Multiplication=Matrix(K*u)
  Lens 4 : Gain  Gain=TLense(:,:,4)^-1  Multiplication=Matrix(K*u)
  Beam Para.s into Transport : Outport
  wires:
  Lens 1/1 -> Beam Para.s into Transport/1
  Distance 1/1 -> Lens 1/1
  Lens 2/1 -> Distance 1/1
  Distance 2/1 -> Lens 2/1
  Lens 3/1 -> Distance 2/1
  Distance 3/1 -> Lens 3/1
  Lens 4/1 -> Distance 3/1
  Beam Para.s Out of Transport/1 -> Lens 4/1

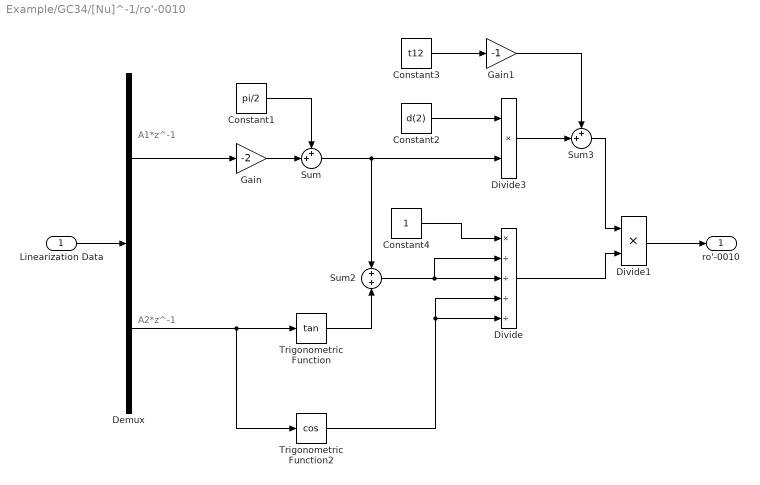
== system Example/GC34/[Nu]^-1/ro'-0010 ==
  note: A1*z^-1
  note: A2*z^-1
  Linearization Data : Inport
  Constant1 : Constant  Value=pi/2
  Constant2 : Constant  Value=d(2)
  Constant3 : Constant  Value=t12
  Constant4 : Constant
  Demux : Demux  Outputs=2
  Divide : Product  Inputs=*////
  Divide1 : Product  Inputs=**
  Divide3 : Product  Inputs=**
  Gain : Gain  Gain=-2
  Gain1 : Gain  Gain=-1
  Sum : Sum  Inputs=++|
  Sum2 : Sum  Inputs=+|+
  Sum3 : Sum  Inputs=++|
  Trigonometric Function : Trigonometry  Operator=tan
  Trigonometric Function2 : Trigonometry  Operator=cos
  ro'-0010 : Outport
  wires:
  Constant4/1 -> Divide/1
  Trigonometric Function2/1 -> Divide/5, Divide/4
  Sum3/1 -> Divide1/1
  Divide3/1 -> Sum3/2
  Gain1/1 -> Sum3/1
  Constant3/1 -> Gain1/1
  Constant2/1 -> Divide3/1
  Divide/1 -> Divide1/2
  Divide1/1 -> ro'-0010/1
  Sum2/1 -> Divide/3, Divide/2
  Demux/2 -> Trigonometric Function/1, Trigonometric Function2/1
  Trigonometric Function/1 -> Sum2/2
  Sum/1 -> Divide3/2, Sum2/1
  Constant1/1 -> Sum/1
  Gain/1 -> Sum/2
  Demux/1 -> Gain/1
  Linearization Data/1 -> Demux/1

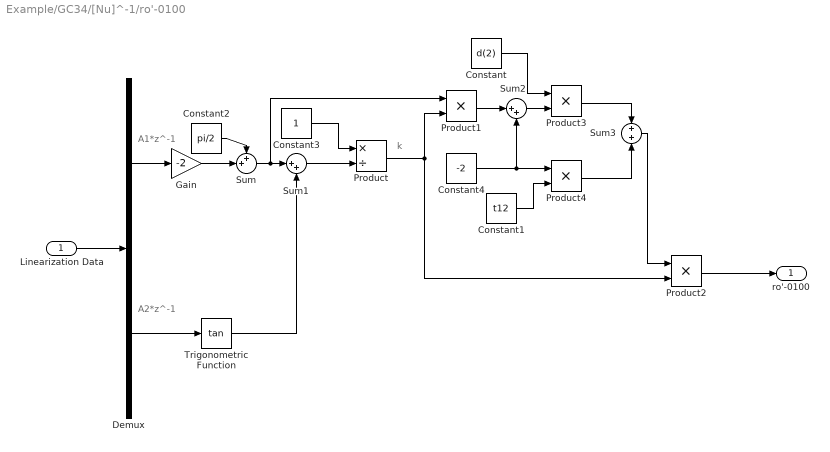
== system Example/GC34/[Nu]^-1/ro'-0100  ==
  note: A1*z^-1
  note: A2*z^-1
  note: k
  Linearization Data : Inport
  Constant : Constant  Value=d(2)
  Constant1 : Constant  Value=t12
  Constant2 : Constant  Value=pi/2
  Constant3 : Constant
  Constant4 : Constant  Value=-2
  Demux : Demux  Outputs=2
  Gain : Gain  Gain=-2
  Product : Product  Inputs=*/
  Product{1..4} (4 alike) : Product  Inputs=**
  Sum : Sum  Inputs=++|
  Sum1 : Sum  Inputs=|++
  Sum2 : Sum  Inputs=|++
  Sum3 : Sum  Inputs=+|+
  Trigonometric Function : Trigonometry  Operator=tan
  ro'-0100 : Outport
  wires:
  Product2/1 -> ro'-0100/1
  Sum3/1 -> Product2/1
  Product3/1 -> Sum3/1
  Product4/1 -> Sum3/2
  Constant1/1 -> Product4/2
  Constant/1 -> Product3/1
  Sum2/1 -> Product3/2
  Constant4/1 -> Sum2/2, Product4/1
  Product1/1 -> Sum2/1
  Sum1/1 -> Product/2
  Sum/1 -> Sum1/1, Product1/1
  Product/1 -> Product2/2, Product1/2
  Constant3/1 -> Product/1
  Trigonometric Function/1 -> Sum1/2
  Demux/2 -> Trigonometric Function/1
  Gain/1 -> Sum/2
  Demux/1 -> Gain/1
  Constant2/1 -> Sum/1
  Linearization Data/1 -> Demux/1

== system Example/Virtual Plant1/OP1 to OP2/Beam Pass 1 ==
  Optical Plane 1 Parameters : Inport
  Demux : Demux  Outputs=2
  Mux : Mux  Inputs=2
  Sine : Trigonometry
  Snell Ratio : Gain  Gain=n_FS/n_BS
  Sum : Sum  Inputs=|++
  Sum1 : Sum  Inputs=|+-
  Tangent : Trigonometry  Operator=tan
  Thickness Offset 1 : Gain  Gain=D(1)*cos(Beta(1))
  Thickness Offset 2 : Constant  Value=D(1)*sin(Beta(1))
  'l6 : Outport
  wires:
  Thickness Offset 2/1 -> Sum1/2
  Thickness Offset 1/1 -> Sum1/1
  Tangent/1 -> Thickness Offset 1/1
  Sine/1 -> Snell Ratio/1
  Snell Ratio/1 -> Tangent/1
  Demux/2 -> Mux/2, Sine/1
  Sum1/1 -> Sum/2
  Sum/1 -> Mux/1
  Demux/1 -> Sum/1
  Mux/1 -> 'l6/1
  Optical Plane 1 Parameters/1 -> Demux/1

== system Example/Virtual Plant1/OP1 to OP2/Beam Pass 2 ==
  l6' : Inport
  Demux : Demux  Outputs=2
  Mux : Mux  Inputs=2
  Sine : Trigonometry
  Snell Ratio : Gain  Gain=n_FS/n_BS
  Sum : Sum  Inputs=|++
  Sum1 : Sum  Inputs=|+-
  Tangent : Trigonometry  Operator=tan
  Thickness Offset 1 : Gain  Gain=D(2)*cos(Beta(2))
  Thickness Offset 2 : Constant  Value=D(2)*sin(Beta(2))
  'l7 : Outport
  wires:
  l6'/1 -> Demux/1
  Mux/1 -> 'l7/1
  Demux/1 -> Sum/1
  Sum/1 -> Mux/1
  Sum1/1 -> Sum/2
  Demux/2 -> Sine/1, Mux/2
  Snell Ratio/1 -> Tangent/1
  Sine/1 -> Snell Ratio/1
  Tangent/1 -> Thickness Offset 1/1
  Thickness Offset 1/1 -> Sum1/1
  Thickness Offset 2/1 -> Sum1/2

== system Example/Virtual Plant1/OP1 to Sensors 1&2/Beam Reflection 1 ==
  "[OP1]" : Inport
  Constant : Constant  Value=pi/2
  Constant1 : Constant  Value=-2*Beta(1)
  Demux : Demux  Outputs=2
  Gain : Gain  Gain=tan(Beta(1))
  Mux : Mux  Inputs=2
  Sum : Sum  Inputs=+++
  Reflected Beam : Outport
  wires:
  Sum/1 -> Mux/2
  Constant/1 -> Sum/3
  Demux/2 -> Sum/2
  Constant1/1 -> Sum/1
  Gain/1 -> Mux/1
  Mux/1 -> Reflected Beam/1
  Demux/1 -> Gain/1
  "[OP1]"/1 -> Demux/1

== system Example/Virtual Plant1/OP1 to Sensors 1&2/Beam Reflection 2 ==
  "[OP1]" : Inport
  Constant : Constant  Value=pi/2
  Constant1 : Constant  Value=-2*Beta(2)
  Demux : Demux  Outputs=2
  Gain : Gain  Gain=tan(Beta(2))
  Mux : Mux  Inputs=2
  Sum : Sum  Inputs=+++
  Reflected Beam : Outport
  wires:
  "[OP1]"/1 -> Demux/1
  Demux/1 -> Gain/1
  Mux/1 -> Reflected Beam/1
  Gain/1 -> Mux/1
  Demux/2 -> Sum/2
  Constant/1 -> Sum/3
  Sum/1 -> Mux/2
  Constant1/1 -> Sum/1

== system Example/Virtual Plant1/OP2 to Sensors 3&4/Beam Reflection 3 ==
  "[OP2]" : Inport
  Constant : Constant  Value=pi/2
  Constant1 : Constant  Value=-2*Beta(3)
  Demux : Demux  Outputs=2
  Gain : Gain  Gain=tan(Beta(3))
  Mux : Mux  Inputs=2
  Sum : Sum  Inputs=+++
  Reflected Beam : Outport
  wires:
  Sum/1 -> Mux/2
  Constant/1 -> Sum/3
  Demux/2 -> Sum/2
  Gain/1 -> Mux/1
  Mux/1 -> Reflected Beam/1
  Demux/1 -> Gain/1
  "[OP2]"/1 -> Demux/1
  Constant1/1 -> Sum/1

== system Example/Virtual Plant1/OP2 to Sensors 3&4/Beam Reflection 4 ==
  "[OP2]*l(9)" : Inport
  Constant : Constant  Value=pi/2
  Constant1 : Constant  Value=-2*Beta(4)
  Demux : Demux  Outputs=2
  Gain : Gain  Gain=tan(Beta(4))
  Mux : Mux  Inputs=2
  Sum : Sum  Inputs=+++
  Reflected Beam : Outport
  wires:
  "[OP2]*l(9)"/1 -> Demux/1
  Demux/1 -> Gain/1
  Mux/1 -> Reflected Beam/1
  Gain/1 -> Mux/1
  Demux/2 -> Sum/2
  Constant/1 -> Sum/3
  Sum/1 -> Mux/2
  Constant1/1 -> Sum/1

== matlab function Example/PLANT/MATLAB Function1 ==
  data: SocketID input; ErrorReturn output; PositionerID input; AbsolutePosition input
function ErrorReturn = Move_Actuator(SocketID, PositionerID, AbsolutePosition)
%#codegen
%Recieves Absolute Position and which positioner, Reports error codes

[errorCode]=GroupMoveAbsolute(SocketID, PositionerID, AbsolutePosition);


ErrorReturn = errorCode;

== matlab function Example/PLANT/MATLAB Function ==
  data: SocketID input; ErrorReturn output; PositionerID input; AbsolutePosition input
function ErrorReturn = Move_Actuator(SocketID, PositionerID, AbsolutePosition)
%#codegen
%Recieves Absolute Position and which positioner, Reports error codes

[errorCode]=GroupMoveAbsolute(SocketID, PositionerID, AbsolutePosition);


ErrorReturn = errorCode;

== matlab function Example/PLANT/MATLAB Function2 ==
  data: SocketID input; ErrorReturn output; PositionerID input; AbsolutePosition input
function ErrorReturn = Move_Actuator(SocketID, PositionerID, AbsolutePosition)
%#codegen
%Recieves Absolute Position and which positioner, Reports error codes

[errorCode]=GroupMoveAbsolute(SocketID, PositionerID, AbsolutePosition);


ErrorReturn = errorCode;

== matlab function Example/PLANT/MATLAB Function3 ==
  data: SocketID input; ErrorReturn output; PositionerID input; AbsolutePosition input
function ErrorReturn = Move_Actuator(SocketID, PositionerID, AbsolutePosition)
%#codegen
%Recieves Absolute Position and which positioner, Reports error codes

[errorCode]=GroupMoveAbsolute(SocketID, PositionerID, AbsolutePosition);


ErrorReturn = errorCode;
